simulink model "parent"  (R2025b)
settings: Solver=FixedStepDiscrete  StartTime=0.0  StopTime=inf  RelTol=1e-3
settings Model: PacingRate=0.500000  Creator=matthewkeller  LastModifiedBy=ryanj
settings OptimizationCC: DefaultParameterBehavior=Inlined  EnhancedBackFolding=on  PassReuseOutputArgsThreshold=0.0  ZeroExternalMemoryAtStartup=off  ZeroInternalMemoryAtStartup=off  OptimizeBlockOrder=speed  DifferentSizesBufferReuse=on  OptimizationCustomize=off
settings DebuggingCC: ParameterTunabilityLossMsg=error
settings SFSimCC: MATLABDynamicMemAlloc=off
settings RTWCC: SystemTargetFile=rtmaps.tlc  TemplateMakefile=rtmaps_default_tmf  RetainRTWFile=on  TargetLang=C++  Description=Generate an RTMaps component embedding the model
settings CodeAppCC: ForceParamTrailComments=on  OperatorAnnotations=on
settings STFCustomTargetCC: SystemTargetFile=rtmaps.tlc  TargetLangStandard=C++11 (ISO)  ModelReferenceCompliant=off  CombineOutputUpdateFcns=on  CodeInterfacePackaging=C++ class  SubcomponentCodeInterfacePackaging=C++ class  CPPClassGenCompliant=on  GRTInterface=off  RTMaps_GRTInterface=0  RTMaps_MultiInstanceCode=1  RTMAPS_BOARD=vc.net2022_x64  RTMaps_CombineOutputUpdateFcns=1  RTMAPS_OS=vc.net2022  RTMAPS_ARCH=x86_64  DisplayOptimOptions=off  RTMAPS_SDKDIR=C:\Program Files\Intempora\RTMaps 4  CustomFileTemplate=rtmaps_file_process.tlc  RTMaps_GenerateAllocFcn=0  RTMaps_MatFileLogging=0  RTMaps_GenerateERTSFunction=0  RTMaps_IntegerCode=0
settings GRTTargetCC: TargetLangStandard=C++11 (ISO)  ModelReferenceCompliant=off  ParMdlRefBuildCompliant=off  CompOptLevelCompliant=off  MatFileLogging=off  CodeInterfacePackaging=C++ class  SubcomponentCodeInterfacePackaging=C++ class  UseToolchainInfoCompliant=off

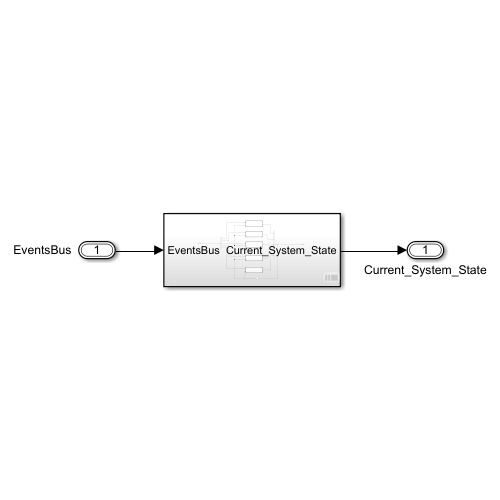
[thumbnail: Simulink's stored preview of the top-level diagram]
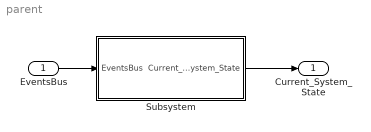
== system parent ==
  EventsBus : Inport  OutDataTypeStr=Bus: EventsBus
  Subsystem : Subsystem
  Current_System_State : Outport  OutDataTypeStr=Bus: CurrentStateBus
  wires:
  EventsBus/1 -> Subsystem/1(EventsBus)
  Subsystem/1(Current_System_State) -> Current_System_State/1

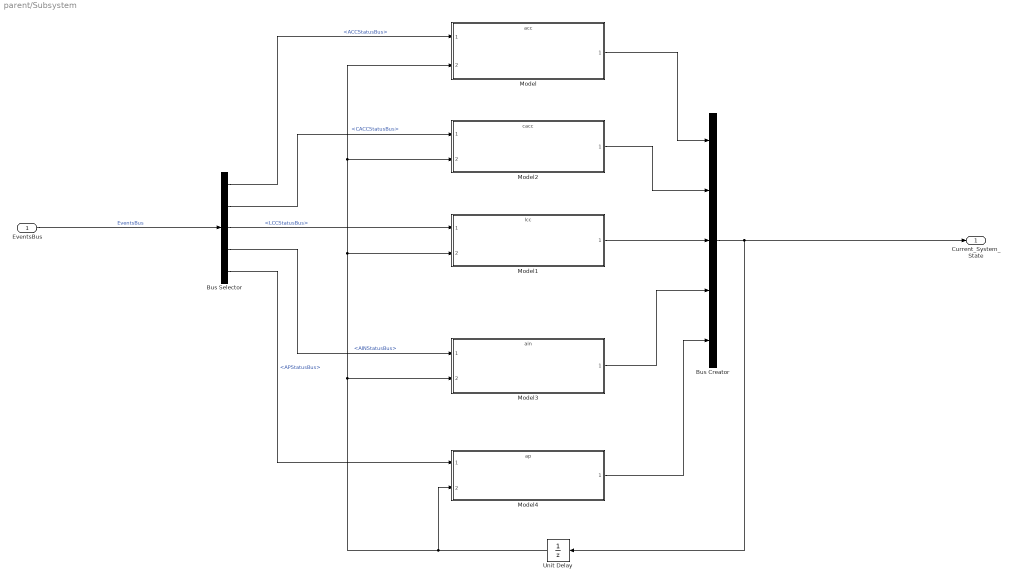
== system parent/Subsystem ==
  EventsBus : Inport  OutDataTypeStr=Bus: EventsBus
  Bus Creator : BusCreator  Inputs=5  OutDataTypeStr=Bus: CurrentStateBus
      settings: InheritFromInputs=off
  Bus Selector : BusSelector  OutputSignals=ACCStatusBus,CACCStatusBus,LCCStatusBus,AINStatusBus,APStatusBus
  Model : ModelReference  ModelNameDialog=acc  SimulationMode=Normal  ModelReferenceVersion=2.0
  Model1 : ModelReference  ModelNameDialog=lcc  SimulationMode=Normal  ModelReferenceVersion=1.41
  Model2 : ModelReference  ModelNameDialog=cacc  SimulationMode=Normal  ModelReferenceVersion=1.53
  Model3 : ModelReference  ModelNameDialog=ain  SimulationMode=Normal  ModelReferenceVersion=1.50
  Model4 : ModelReference  ModelNameDialog=ap  SimulationMode=Normal  ModelReferenceVersion=1.41
  Unit Delay : UnitDelay  SampleTime=-1  HasFrameUpgradeWarning=on
  Current_System_State : Outport
  wires:
  Bus Selector/4 -> Model3/1  "<AINStatusBus>"
  Bus Selector/3 -> Model1/1  "<LCCStatusBus>"
  Bus Selector/1 -> Model/1  "<ACCStatusBus>"
  Bus Selector/2 -> Model2/1  "<CACCStatusBus>"
  Bus Selector/5 -> Model4/1  "<APStatusBus>"
  EventsBus/1 -> Bus Selector/1  "EventsBus"
  Bus Creator/1 -> Current_System_State/1, Unit Delay/1
  Model/1 -> Bus Creator/1
  Model2/1 -> Bus Creator/2
  Model1/1 -> Bus Creator/3
  Model3/1 -> Bus Creator/4
  Model4/1 -> Bus Creator/5
  Unit Delay/1 -> Model3/2, Model/2, Model2/2, Model1/2, Model4/2
